simulink model "sampleModel1975"  (R2023a)
settings: Solver=VariableStepAuto  StartTime=0.0  StopTime=10.0  RelTol=1e-3
libraries: hdlsllib x3, simulink x1
settings Model: Creator=user1  LastModifiedBy=user1

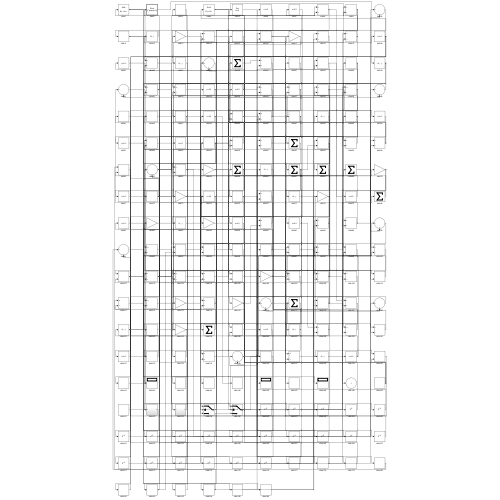
[thumbnail: Simulink's stored preview of the top-level diagram]
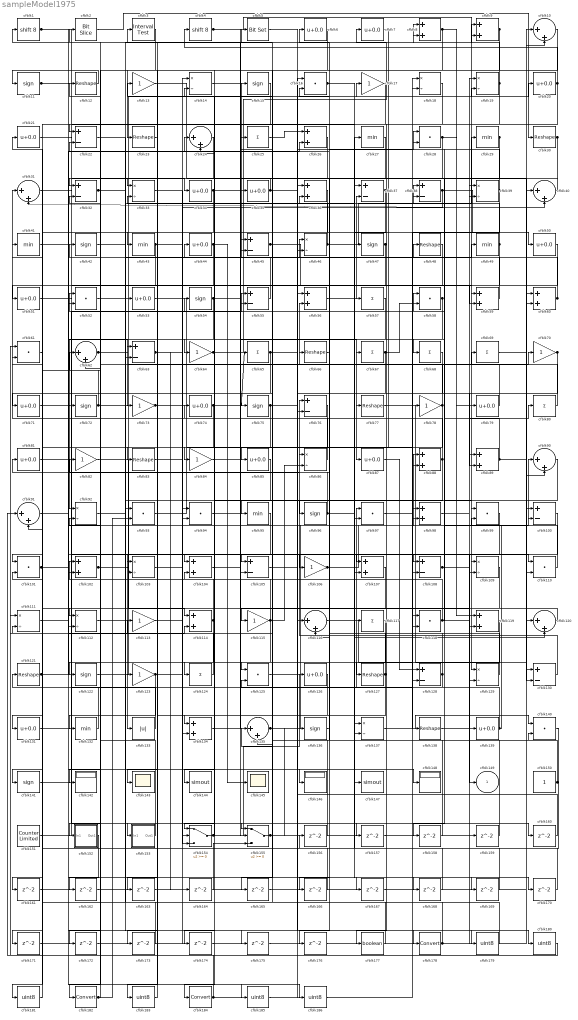
== system sampleModel1975 ==
  cfblk1 : ArithShift  BitShiftNumber=8
  cfblk{10,24,31,40,62,90..91,116,120,135} (10 alike) : Sum  Inputs=|++
  cfblk{22,32,37..38,45,55,63,76,100,105,108,128,130} (13 alike) : Sum  Inputs=+-
  cfblk{16,28,52,58,61,93..94,97,99,101,110,118,125,140} (14 alike) : DotProduct  OutDataTypeStr=Inherit: Inherit via internal rule
  cfblk{8..9,26,36,56,59..60,88..89,98,102,104,107,114,119,134} (16 alike) : Sum
  cfblk{14,18..19,33,39,46,86,92,103,109,111..112,129,137} (14 alike) : Product  Inputs=*/  RndMeth=Zero  SaturateOnIntegerOverflow=on
  cfblk{13,17,64,70,73,78,82,84,106,113,115,123} (12 alike) : Gain
  cfblk{11,15,42,47,54,72,75,96,122,136,141} (11 alike) : Signum
  cfblk{25,57,65,67..69,80,117,124} (9 alike) : Sum  Inputs=+
  cfblk{12,23,30,48,66,77,83,121,127,138} (10 alike) : Reshape
  cfblk{6..7,20..21,34..35,44,50..51,53,71,74,79,81,85,87,126,131,139} (19 alike) : Bias  Bias=0.0  SaturateOnIntegerOverflow=off
  cfblk{27,29,41,43,49,95,132} (7 alike) : MinMax
  cfblk133 : Abs  SaturateOnIntegerOverflow=off
  cfblk142 : Display
  cfblk143 : Scope
  cfblk144 : ToWorkspace  VariableName=simout  SaveFormat=Timeseries  SampleTime=-1
  cfblk145 : Scope
  cfblk146 : Display
  cfblk147 : ToWorkspace  VariableName=simout  SaveFormat=Timeseries  SampleTime=-1
  cfblk148 : Display
  cfblk150 : Constant  SampleTime=-1
  cfblk151 : hdlsllib/Sources/Counter Limited  uplimit=7  tsamp=-1
  cfblk152 : Subsystem
      settings: LibrarySourceBlock=|
      | hdlsllib/Ports &
      | Subsystems/Subsystem
  cfblk153 : Subsystem
      settings: LibrarySourceBlock=|
      | hdlsllib/Ports &
      | Subsystems/Subsystem
  cfblk154 : Switch  SaturateOnIntegerOverflow=off  InputSameDT=off
  cfblk155 : Switch  SaturateOnIntegerOverflow=off  InputSameDT=off
  cfblk{156..176} (21 alike) : Delay  SampleTime=1
  cfblk177 : DataTypeConversion  OutDataTypeStr=boolean  SaturateOnIntegerOverflow=off  RndMeth=Floor
  cfblk178 : DataTypeConversion  SaturateOnIntegerOverflow=off  RndMeth=Floor
  cfblk{179..181,183,185..186} (6 alike) : DataTypeConversion  OutDataTypeStr=uint8  SaturateOnIntegerOverflow=off  RndMeth=Floor
  cfblk182 : DataTypeConversion  SaturateOnIntegerOverflow=off  RndMeth=Floor
  cfblk184 : DataTypeConversion  SaturateOnIntegerOverflow=off  RndMeth=Floor
  cfblk2 : hdlsllib/Logic and Bit Operations/Bit Slice  lidx=7  ridx=0
  cfblk3 : hdlsllib/Logic and Bit Operations/Interval Test  IntervalClosedRight=on  uplimit=0.5  IntervalClosedLeft=on  lowlimit=-0.5  OutDataTypeStr=boolean
  cfblk4 : ArithShift  BitShiftNumber=8
  cfblk5 : simulink/Logic and Bit Operations/Bit Set  iBit=0
      settings: LibrarySourceBlock=|
      | hdlsllib/Logic and Bit
      | Operations/Bit Set
  cfblk149 : Outport  VectorParamsAs1DForOutWhenUnconnected=off
  wires:
  cfblk112/1 -> cfblk17/1
  cfblk64/1 -> cfblk7/1, cfblk110/2
  cfblk87/1 -> cfblk128/1
  cfblk7/1 -> cfblk143/1
  cfblk4/1 -> cfblk129/1, cfblk59/2, cfblk8/2
  cfblk60/1 -> cfblk15/1, cfblk24/1
  cfblk86/1 -> cfblk31/1
  cfblk59/1 -> cfblk48/1
  cfblk67/1 -> cfblk87/1, cfblk107/1, cfblk76/2, cfblk58/2
  cfblk30/1 -> cfblk109/1, cfblk63/2
  cfblk11/1 -> cfblk57/1, cfblk169/1
  cfblk56/1 -> cfblk37/2
  cfblk2/1 -> cfblk30/1
  cfblk79/1 -> cfblk56/2
  cfblk35/1 -> cfblk33/1, cfblk28/1
  cfblk51/1 -> cfblk105/1
  cfblk1/1 -> cfblk104/1, cfblk63/1, cfblk186/1
  cfblk73/1 -> cfblk95/1, cfblk138/1
  cfblk130/1 -> cfblk76/1
  cfblk55/1 -> cfblk35/1
  cfblk122/1 -> cfblk27/1
  cfblk31/1 -> cfblk59/1
  cfblk71/1 -> cfblk153/1(In1)
  cfblk21/1 -> cfblk34/1
  cfblk151/1 -> cfblk55/1
  cfblk103/1 -> cfblk69/1
  cfblk77/1 -> cfblk129/2
  cfblk20/1 -> cfblk22/1, cfblk4/1, cfblk127/1, cfblk101/1
  cfblk36/1 -> cfblk43/1
  cfblk58/1 -> cfblk92/1, cfblk52/2
  cfblk6/1 -> cfblk84/1
  cfblk53/1 -> cfblk137/1
  cfblk45/1 -> cfblk25/1, cfblk147/1
  cfblk141/1 -> cfblk90/1
  cfblk82/1 -> cfblk114/1
  cfblk18/1 -> cfblk184/1
  cfblk75/1 -> cfblk154/3, cfblk180/1
  cfblk100/1 -> cfblk133/1
  cfblk115/1 -> cfblk82/1, cfblk86/2, cfblk134/2
  cfblk93/1 -> cfblk96/1
  cfblk96/1 -> cfblk21/1, cfblk168/1
  cfblk62/1 -> cfblk54/1, cfblk8/1, cfblk47/1
  cfblk120/1 -> cfblk115/1
  cfblk78/1 -> cfblk45/1, cfblk85/1, cfblk137/2
  cfblk10/1 -> cfblk23/1
  cfblk135/1 -> cfblk88/1, cfblk78/1
  cfblk72/1 -> cfblk66/1, cfblk148/1, cfblk41/1
  cfblk44/1 -> cfblk122/1, cfblk145/1
  cfblk110/1 -> cfblk38/1
  cfblk12/1 -> cfblk11/1
  cfblk25/1 -> cfblk26/1
  cfblk118/1 -> cfblk38/2, cfblk44/1, cfblk130/2
  cfblk61/1 -> cfblk131/1
  cfblk94/1 -> cfblk20/1
  cfblk9/1 -> cfblk24/2, cfblk165/1
  cfblk57/1 -> cfblk77/1
  cfblk84/1 -> cfblk105/2
  cfblk128/1 -> cfblk42/1, cfblk125/2
  cfblk138/1 -> cfblk19/1
  cfblk125/1 -> cfblk10/1
  cfblk32/1 -> cfblk2/1, cfblk154/2
  cfblk54/1 -> cfblk73/1, cfblk46/1, cfblk119/2, cfblk112/1
  cfblk47/1 -> cfblk83/1, cfblk154/1
  cfblk49/1 -> cfblk33/2, cfblk94/2, cfblk116/2
  cfblk69/1 -> cfblk90/2
  cfblk85/1 -> cfblk124/1
  cfblk40/1 -> cfblk32/1
  cfblk139/1 -> cfblk97/1, cfblk99/2
  cfblk27/1 -> cfblk106/1
  cfblk39/1 -> cfblk68/1, cfblk16/2, cfblk118/2
  cfblk116/1 -> cfblk128/2
  cfblk131/1 -> cfblk117/1
  cfblk23/1 -> cfblk103/1
  cfblk153/1(Out1) -> cfblk102/1
  cfblk46/1 -> cfblk29/1, cfblk14/2
  cfblk150/1 -> cfblk6/1, cfblk13/1, cfblk140/2
  cfblk134/1 -> cfblk49/1
  cfblk121/1 -> cfblk86/1, cfblk114/2
  cfblk80/1 -> cfblk52/1
  cfblk89/1 -> cfblk60/2, cfblk28/2
  cfblk129/1 -> cfblk22/2
  cfblk117/1 -> cfblk135/2
  cfblk52/1 -> cfblk53/1
  cfblk114/1 -> cfblk92/2, cfblk152/1(In1)
  cfblk29/1 -> cfblk108/1, cfblk112/2
  cfblk15/1 -> cfblk55/2
  cfblk48/1 -> cfblk51/1
  cfblk70/1 -> cfblk89/2, cfblk107/2
  cfblk104/1 -> cfblk70/1
  cfblk76/1 -> cfblk144/1
  cfblk26/1 -> cfblk64/1
  cfblk106/1 -> cfblk10/2, cfblk120/2
  cfblk108/1 -> cfblk149/1, cfblk58/1
  cfblk17/1 -> cfblk71/1
  cfblk13/1 -> cfblk100/1
  cfblk101/1 -> cfblk98/1, cfblk26/2
  cfblk124/1 -> cfblk113/1
  cfblk65/1 -> cfblk170/1, cfblk181/1
  cfblk63/1 -> cfblk110/1, cfblk164/1
  cfblk22/1 -> cfblk99/1
  cfblk38/1 -> cfblk130/1, cfblk31/2
  cfblk37/1 -> cfblk132/1, cfblk155/2
  cfblk107/1 -> cfblk125/1
  cfblk83/1 -> cfblk19/2
  cfblk95/1 -> cfblk102/2
  cfblk43/1 -> cfblk142/1, cfblk155/1
  cfblk113/1 -> cfblk14/1
  cfblk16/1 -> cfblk50/1, cfblk109/2
  cfblk50/1 -> cfblk97/2
  cfblk137/1 -> cfblk140/1
  cfblk123/1 -> cfblk40/2, cfblk172/1
  cfblk127/1 -> cfblk81/1, cfblk174/1
  cfblk155/1 -> cfblk39/2, cfblk136/1, cfblk139/1
  cfblk133/1 -> cfblk121/1
  cfblk154/1 -> cfblk126/1, cfblk74/1
  cfblk5/1 -> cfblk178/1
  cfblk97/1 -> cfblk108/2
  cfblk74/1 -> cfblk65/1, cfblk171/1
  cfblk34/1 -> cfblk141/1, cfblk9/1
  cfblk98/1 -> cfblk80/1
  cfblk33/1 -> cfblk98/2
  cfblk3/1 -> cfblk182/1
  cfblk8/1 -> cfblk123/1, cfblk119/1
  cfblk102/1 -> cfblk103/2, cfblk36/2, cfblk100/2
  cfblk14/1 -> cfblk67/1
  cfblk132/1 -> cfblk111/2
  cfblk81/1 -> cfblk146/1
  cfblk28/1 -> cfblk45/2, cfblk79/1
  cfblk19/1 -> cfblk75/1, cfblk9/2
  cfblk24/1 -> cfblk72/1
  cfblk88/1 -> cfblk62/2, cfblk134/1
  cfblk140/1 -> cfblk156/1
  cfblk156/1 -> cfblk104/2
  cfblk105/1 -> cfblk157/1
  cfblk157/1 -> cfblk89/1
  cfblk90/1 -> cfblk158/1
  cfblk158/1 -> cfblk1/1
  cfblk159/1 -> cfblk111/1
  cfblk92/1 -> cfblk160/1
  cfblk160/1 -> cfblk16/1
  cfblk109/1 -> cfblk161/1
  cfblk161/1 -> cfblk36/1
  cfblk152/1(Out1) -> cfblk162/1
  cfblk162/1 -> cfblk56/1
  cfblk99/1 -> cfblk163/1
  cfblk163/1 -> cfblk60/1
  cfblk164/1 -> cfblk155/3
  cfblk165/1 -> cfblk40/1
  cfblk66/1 -> cfblk166/1
  cfblk166/1 -> cfblk135/1
  cfblk41/1 -> cfblk167/1
  cfblk167/1 -> cfblk39/1
  cfblk168/1 -> cfblk61/2
  cfblk169/1 -> cfblk37/1
  cfblk170/1 -> cfblk32/2
  cfblk171/1 -> cfblk120/1
  cfblk172/1 -> cfblk94/1
  cfblk119/1 -> cfblk173/1
  cfblk173/1 -> cfblk62/1
  cfblk174/1 -> cfblk118/1
  cfblk42/1 -> cfblk175/1
  cfblk175/1 -> cfblk116/1
  cfblk136/1 -> cfblk176/1
  cfblk176/1 -> cfblk88/2
  cfblk68/1 -> cfblk177/1
  cfblk177/1 -> cfblk5/1
  cfblk178/1 -> cfblk159/1, cfblk101/2
  cfblk91/1 -> cfblk179/1
  cfblk179/1 -> cfblk93/1
  cfblk180/1 -> cfblk91/1
  cfblk181/1 -> cfblk91/2
  cfblk182/1 -> cfblk12/1, cfblk93/2
  cfblk126/1 -> cfblk183/1
  cfblk183/1 -> cfblk3/1
  cfblk184/1 -> cfblk46/2, cfblk61/1
  cfblk111/1 -> cfblk185/1
  cfblk185/1 -> cfblk18/1
  cfblk186/1 -> cfblk18/2

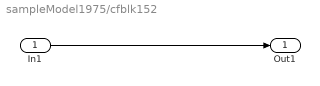
== system sampleModel1975/cfblk152 ==
  In1 : Inport
  Out1 : Outport
  wires:
  In1/1 -> Out1/1

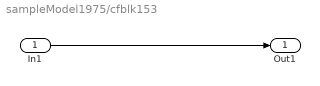
== system sampleModel1975/cfblk153 ==
  In1 : Inport
  Out1 : Outport
  wires:
  In1/1 -> Out1/1
